simulink model "vertical_channel"  (R2015a)
settings: Solver=ode45  StartTime=0.0  StopTime=10.0  MaxStep=0.1  RelTol=1e-3
undefined symbols (not defined in the file): Zw
settings Model: FPTRunName=Active  ModifiedByFormat=The MathWorks Inc.  CovSFcnEnable=off  Creator=The MathWorks Inc.  LastModifiedBy=The MathWorks Inc.
settings ConfigSet: ConfigType=Model
settings SolverCC: Priority=auto
settings DataIOCC: SaveOutput=off  SaveTime=off  SignalLoggingName=vertical_channel
settings OptimizationCC: InlineParams=on  InlineParamsCompatibleMode=off  ExpressionDepthLimit=2147483647  InitFltsAndDblsToZero=on  ForceBlockIOInitOptimize=off  EvaledLifeSpan=1  SimCompilerOptimization=Off
settings DebuggingCC: SaveWithParameterizedLinksMsg=none  UnderspecifiedInitializationDetection=Classic  MergeDetectMultiDrivingBlocksExec=none  SignalResolutionControl=TryResolveAllWithWarning  SolverPrmCheckMsg=warning  MultiTaskDSMMsg=warning  MultiTaskCondExecSysMsg=none  FcnCallInpInsideContextMsg=UseLocalSettings  AllowSymbolicDim=off  StateNameClashWarn=warning  SFMismatchInSimAndRtwBecauseOfMissingDataTypeDiag=warning
settings RTWCC: EnableTagging=off  RTWCompilerOptimization=Off
settings CodeAppCC: ParameterTuningSideEffectCode=Output function  AllmanStyle=off
settings GRTTargetCC: TargetFcnLib=ansi_tfl_tmw.mat  CombineOutputUpdateFcns=off  EnableShiftOperators=off  PortableWordSizesTransition=off  GenerateErtSFunctionTransition=off  CreateSILPILBlockTransition=None  CodeProfilingSaveOptionsTransition=SummaryOnly  CodeExecutionProfilingTransition=off  CodeProfilingInstrumentationTransition=off  CodeExecutionProfileVariableTransition=executionProfile  GRTInterface=on

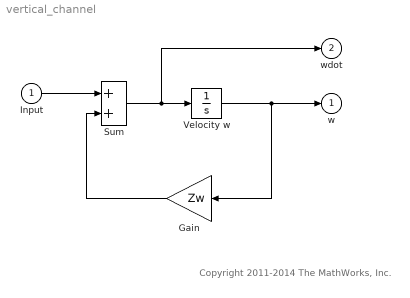
== system vertical_channel ==
  note: Copyright 2011-2014 The MathWorks, Inc.
  Input : Inport  IOType=none  Commented=off  StatePerturbationForJacobian=1.0e-05
  Gain : Gain  IOType=none  Commented=off  StatePerturbationForJacobian=1.0e-05  Gain=Zw  SaturateOnIntegerOverflow=on  OutDataTypeStr=Inherit: Same as input  ParamDataTypeStr=Inherit: Same as input
  Sum : Sum  IOType=none  Commented=off  StatePerturbationForJacobian=1.0e-05  SaturateOnIntegerOverflow=on  InputSameDT=on  OutDataTypeStr=Inherit: Same as first input
  Velocity w : Integrator  IOType=none  Commented=off  StatePerturbationForJacobian=1.0e-05
  w : Outport  IOType=none  Commented=off  StatePerturbationForJacobian=1.0e-05
  wdot : Outport  IOType=none  Commented=off  StatePerturbationForJacobian=1.0e-05  Port=2
  wires:
  Input/1 -> Sum/1
  Gain/1 -> Sum/2
  Velocity w/1 -> w/1, Gain/1
  Sum/1 -> Velocity w/1, wdot/1
